simulink model "Redresseur_MLI_3Ph_2021_MLI_abc_s3b"  (R2022b)
settings: Solver=ode8  StartTime=0.0  StopTime=0.1  FixedStep=1e-6  RelTol=1e-3
undefined symbols (not defined in the file): C, Im, inverter_matrix, K, L, R, Ta, Td, Ti, V
libraries: simulink x1
settings Model: Creator=driss  LastModifiedBy=driss
settings RTWCC: GPUComputeCapability=5.0

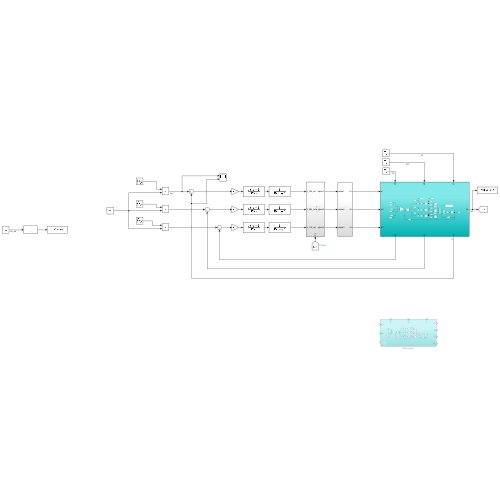
[thumbnail: Simulink's stored preview of the top-level diagram]
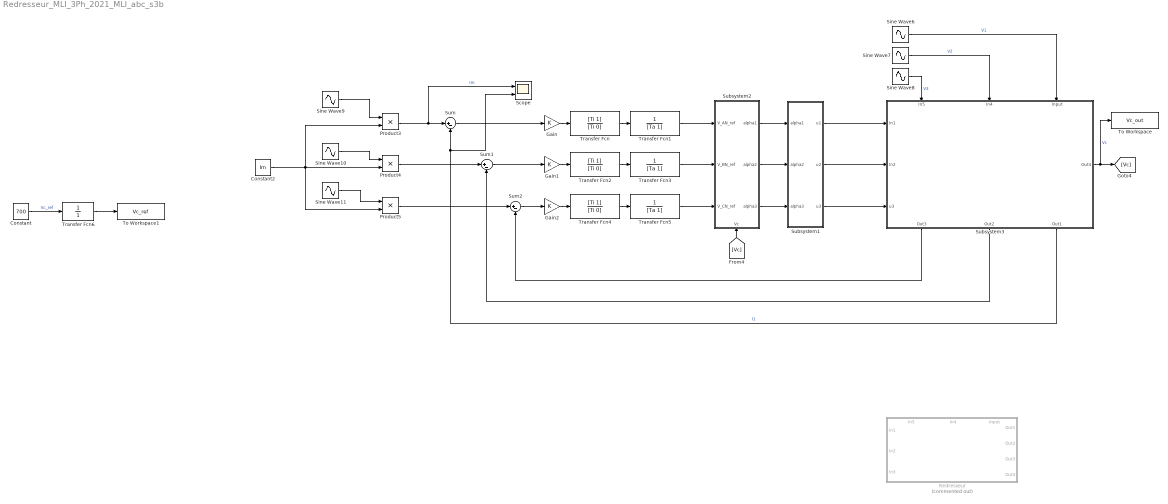
== system Redresseur_MLI_3Ph_2021_MLI_abc_s3b ==
  Constant : Constant  Value=700
  Constant2 : Constant  Value=Im
  Gain : Gain  Gain=K
  Gain1 : Gain  Gain=K
  Gain2 : Gain  Gain=K
  Product3 : Product
  Product4 : Product
  Product5 : Product
  Redresseur : Subsystem  Commented=on
      settings: PortSchema="{\"entries\":[{\"content\":{\"sides\":[{\"content\":{\"connectorIds\":[\"In1\",\"In2\",\"In3\"]},\"type\":\"ConnectorPlacement.EquallySpacedRectSide\",\"uuid\":\"ae9b6999-67aa-4d3c-bad5-5678f4aa6fd1\"},{\"content\":{\"connectorIds\":[\"Out1\",\"Out2\",\"Out3\",\"Out4\"],\"side\":\"RIGHT\"},\"type\":\"ConnectorPlacement.EquallySpacedRectSide\",\"uuid\":\"c2ea9883-df9a-4db0-b590-77b43908e459\"},{\"content\":{\"connectorIds\":[\"In4\",\"In5\",\"In6\"],\"side\":\"TOP\"},\"type\":\"ConnectorPlacement.EquallySpacedRectSide\",\"uuid\":\"cd2a08bf-72f9-4cdd-a271-8309bde71cde\"},{\"content\":{\"side\":\"BOTTOM\"},\"type\":\"ConnectorPlacement.EquallySpacedRectSide\",\"uuid\":\"317f1b40-2736-47c4-82a9-6da6172d899a\"}]},\"type\":\"ConnectorPlacement.EquallySpacedConnector\",\"uuid\":\"e059e48c-1350-41c9-95f4-730b69f1f213\"}],\"packageUris\":[\"http://schema.mathworks.com/mf0/Connector/R2020b\"],\"version\":\"1.0\"}"
  Scope : Scope  NumInputPorts=2
  Sine Wave10 : Sin  Frequency=2*50*pi  Phase=-2*pi/3  SampleTime=0
  Sine Wave11 : Sin  Frequency=2*50*pi  Phase=-4*pi/3  SampleTime=0
  Sine Wave6 : Sin  Amplitude=V*sqrt(2)  Frequency=2*50*pi  SampleTime=0
  Sine Wave7 : Sin  Amplitude=V*sqrt(2)  Frequency=2*50*pi  Phase=-2*pi/3  SampleTime=0
  Sine Wave8 : Sin  Amplitude=V*sqrt(2)  Frequency=2*50*pi  Phase=-4*pi/3  SampleTime=0
  Sine Wave9 : Sin  Frequency=2*50*pi  SampleTime=0
  Subsystem1 : Subsystem
  Subsystem2 : Subsystem
      settings: PortSchema="{\"entries\":[{\"content\":{\"sides\":[{\"content\":{\"connectorIds\":[\"In1\",\"In2\",\"In3\"]},\"type\":\"ConnectorPlacement.EquallySpacedRectSide\",\"uuid\":\"a3c0e225-73b1-4d6d-96ea-a79f2c69e987\"},{\"content\":{\"connectorIds\":[\"Out1\",\"Out2\",\"Out3\"],\"side\":\"RIGHT\"},\"type\":\"ConnectorPlacement.EquallySpacedRectSide\",\"uuid\":\"e47335df-8d84-45b3-8de3-f9ef23b68ce2\"},{\"content\":{\"connectorIds\":[],\"side\":\"TOP\"},\"type\":\"ConnectorPlacement.EquallySpacedRectSide\",\"uuid\":\"700b4ae9-e9d5-449c-823f-e97f4f733a61\"},{\"content\":{\"connectorIds\":[\"In4\"],\"side\":\"BOTTOM\"},\"type\":\"ConnectorPlacement.EquallySpacedRectSide\",\"uuid\":\"4332c11f-da0c-41da-94bc-63e1f62b18da\"}]},\"type\":\"ConnectorPlacement.EquallySpacedConnector\",\"uuid\":\"589f38f2-4ecb-4b26-afeb-66b253271d4e\"}],\"packageUris\":[\"http://schema.mathworks.com/mf0/Connector/R2020b\"],\"version\":\"1.0\"}"
  Subsystem3 : Subsystem
      settings: PortSchema="{\"entries\":[{\"content\":{\"sides\":[{\"content\":{\"connectorIds\":[\"In1\",\"In2\",\"In3\"]},\"type\":\"ConnectorPlacement.EquallySpacedRectSide\",\"uuid\":\"ae9b6999-67aa-4d3c-bad5-5678f4aa6fd1\"},{\"content\":{\"connectorIds\":[\"Out1\"],\"side\":\"RIGHT\"},\"type\":\"ConnectorPlacement.EquallySpacedRectSide\",\"uuid\":\"c2ea9883-df9a-4db0-b590-77b43908e459\"},{\"content\":{\"connectorIds\":[\"In4\",\"In5\",\"In6\"],\"side\":\"TOP\"},\"type\":\"ConnectorPlacement.EquallySpacedRectSide\",\"uuid\":\"cd2a08bf-72f9-4cdd-a271-8309bde71cde\"},{\"content\":{\"connectorIds\":[\"Out2\",\"Out3\",\"Out4\"],\"side\":\"BOTTOM\"},\"type\":\"ConnectorPlacement.EquallySpacedRectSide\",\"uuid\":\"317f1b40-2736-47c4-82a9-6da6172d899a\"}]},\"type\":\"ConnectorPlacement.EquallySpacedConnector\",\"uuid\":\"e059e48c-1350-41c9-95f4-730b69f1f213\"}],\"packageUris\":[\"http://schema.mathworks.com/mf0/Connector/R2020b\"],\"version\":\"1.0\"}"
  Sum : Sum  Inputs=|+-
  Sum1 : Sum  Inputs=|+-
  Sum2 : Sum  Inputs=|+-
  To Workspace : ToWorkspace  VariableName=Vc_out  SaveFormat=Timeseries  SampleTime=-1
  To Workspace1 : ToWorkspace  VariableName=Vc_ref  SaveFormat=Timeseries  SampleTime=-1
  Transfer Fcn : TransferFcn  Numerator=[Ti 1]  Denominator=[Ti 0]
  Transfer Fcn1 : TransferFcn  Denominator=[Ta 1]
  Transfer Fcn2 : TransferFcn  Numerator=[Ti 1]  Denominator=[Ti 0]
  Transfer Fcn3 : TransferFcn  Denominator=[Ta 1]
  Transfer Fcn4 : TransferFcn  Numerator=[Ti 1]  Denominator=[Ti 0]
  Transfer Fcn5 : TransferFcn  Denominator=[Ta 1]
  Transfer Fcn6 : TransferFcn  Denominator=[0 1]
  wires:
  Constant/1 -> Transfer Fcn6/1  "Vc_ref"
  Subsystem2/1(alpha1) -> Subsystem1/1(alpha1)
  Subsystem2/2(alpha2) -> Subsystem1/2(alpha2)
  Subsystem2/3(alpha3) -> Subsystem1/3(alpha3)
  Subsystem1/1(u1) -> Subsystem3/1(In1)
  Subsystem1/2(u2) -> Subsystem3/2(In2)
  Subsystem1/3(u3) -> Subsystem3/3(u3)
  Sine Wave7/1 -> Subsystem3/5(In4)  "V2"
  Sine Wave8/1 -> Subsystem3/4(In5)  "V3"
  Sine Wave6/1 -> Subsystem3/6(Input)  "V1"
  [Vc] -> Subsystem2/4(Vc)
  Subsystem3/1(Out4) -> To Workspace/1, [Vc]  "Vc"
  Sine Wave11/1 -> Product5/1
  Sine Wave10/1 -> Product4/1
  Sine Wave9/1 -> Product3/1
  Constant2/1 -> Product5/2, Product4/2, Product3/2
  Product3/1 -> Scope/1, Sum/1  "Im"
  Product4/1 -> Sum1/1
  Product5/1 -> Sum2/1
  Sum/1 -> Gain/1
  Gain/1 -> Transfer Fcn/1
  Transfer Fcn/1 -> Transfer Fcn1/1
  Transfer Fcn1/1 -> Subsystem2/1(V_AN_ref)
  Transfer Fcn2/1 -> Transfer Fcn3/1
  Gain1/1 -> Transfer Fcn2/1
  Transfer Fcn3/1 -> Subsystem2/2(V_BN_ref)
  Transfer Fcn5/1 -> Subsystem2/3(V_CN_ref)
  Gain2/1 -> Transfer Fcn4/1
  Transfer Fcn4/1 -> Transfer Fcn5/1
  Sum1/1 -> Gain1/1
  Sum2/1 -> Gain2/1
  Subsystem3/2(Out3) -> Sum2/2
  Subsystem3/3(Out2) -> Sum1/2
  Subsystem3/4(Out1) -> Scope/2, Sum/2  "I1"
  Transfer Fcn6/1 -> To Workspace1/1

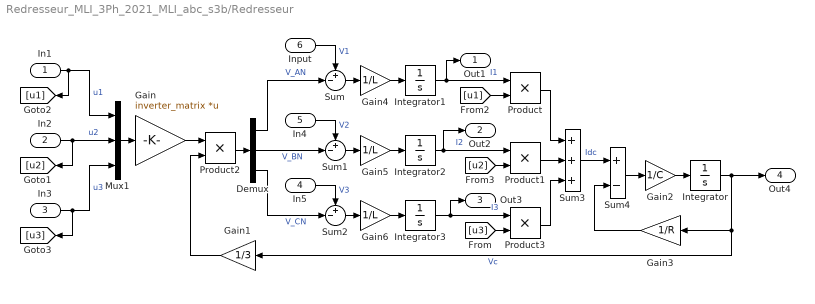
== system Redresseur_MLI_3Ph_2021_MLI_abc_s3b/Redresseur ==
  In1 : Inport
  In2 : Inport  Port=2
  In3 : Inport  Port=3
  In5 : Inport  Port=4
  In4 : Inport  Port=5
  Input : Inport  Port=6
  Demux : Demux  Outputs=3
  Gain : Gain  Gain=inverter_matrix  Multiplication=Matrix(K*u)
  Gain1 : Gain  Gain=1/3
  Gain2 : Gain  Gain=1/C
  Gain3 : Gain  Gain=1/R
  Gain4 : Gain  Gain=1/L
  Gain5 : Gain  Gain=1/L
  Gain6 : Gain  Gain=1/L
  Integrator{,1..3} (4 alike) : Integrator
  Mux1 : Mux  Inputs=3
  Product{,1..3} (4 alike) : Product
  Sum : Sum  Inputs=+-|
  Sum1 : Sum  Inputs=+-|
  Sum2 : Sum  Inputs=+-|
  Sum3 : Sum  Inputs=+++
  Sum4 : Sum  Inputs=+-
  Out1 : Outport
  Out2 : Outport  Port=2
  Out3 : Outport  Port=3
  Out4 : Outport  Port=4
  wires:
  In3/1 -> [u3], Mux1/3  "u3"
  In2/1 -> [u2], Mux1/2  "u2"
  In1/1 -> [u1], Mux1/1  "u1"
  Demux/2 -> Sum1/2  "V_BN"
  Demux/3 -> Sum2/2  "V_CN"
  Demux/1 -> Sum/2  "V_AN"
  Input/1 -> Sum/1  "V1"
  In4/1 -> Sum1/1  "V2"
  In5/1 -> Sum2/1  "V3"
  Sum/1 -> Gain4/1
  Sum1/1 -> Gain5/1
  Sum2/1 -> Gain6/1
  Integrator1/1 -> Out1/1, Product/1  "I1"
  Integrator3/1 -> Out3/1, Product3/1  "I3"
  Integrator2/1 -> Product1/1, Out2/1  "I2"
  Mux1/1 -> Gain/1
  [u3] -> Product3/2
  Product/1 -> Sum3/1
  Product1/1 -> Sum3/2
  Product3/1 -> Sum3/3
  Gain1/1 -> Product2/2
  Gain/1 -> Product2/1
  Sum3/1 -> Sum4/1  "Idc"
  Sum4/1 -> Gain2/1
  Gain2/1 -> Integrator/1
  Integrator/1 -> Out4/1, Gain1/1, Gain3/1  "Vc"
  Gain3/1 -> Sum4/2
  Gain4/1 -> Integrator1/1
  Gain5/1 -> Integrator2/1
  Gain6/1 -> Integrator3/1
  Product2/1 -> Demux/1
  [u1] -> Product/2
  [u2] -> Product1/2

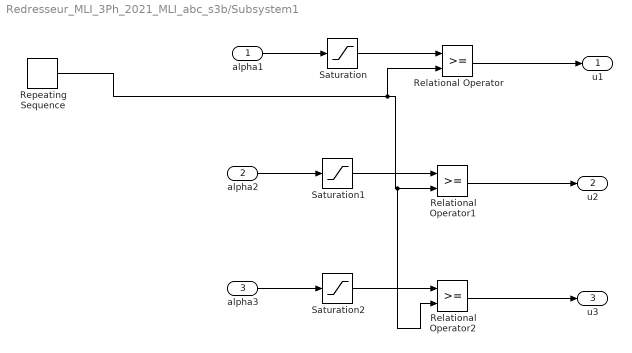
== system Redresseur_MLI_3Ph_2021_MLI_abc_s3b/Subsystem1 ==
  alpha1 : Inport
  alpha2 : Inport  Port=2
  alpha3 : Inport  Port=3
  Relational Operator : RelationalOperator  OutDataTypeStr=boolean  RndMeth=Simplest  InputSameDT=off
  Relational Operator1 : RelationalOperator  OutDataTypeStr=boolean  RndMeth=Simplest  InputSameDT=off
  Relational Operator2 : RelationalOperator  OutDataTypeStr=boolean  RndMeth=Simplest  InputSameDT=off
  Repeating Sequence : simulink/Sources/Repeating Sequence  rep_seq_t=[0 Td/2 Td]  rep_seq_y=[1 0 1]
  Saturation : Saturate  UpperLimit=1  LowerLimit=0
  Saturation1 : Saturate  UpperLimit=1  LowerLimit=0
  Saturation2 : Saturate  UpperLimit=1  LowerLimit=0
  u1 : Outport
  u2 : Outport  Port=2
  u3 : Outport  Port=3
  wires:
  Saturation/1 -> Relational Operator/1
  Relational Operator/1 -> u1/1
  alpha1/1 -> Saturation/1
  Saturation1/1 -> Relational Operator1/1
  Relational Operator1/1 -> u2/1
  alpha2/1 -> Saturation1/1
  Saturation2/1 -> Relational Operator2/1
  Relational Operator2/1 -> u3/1
  alpha3/1 -> Saturation2/1
  Repeating Sequence/1 -> Relational Operator2/2, Relational Operator1/2, Relational Operator/2

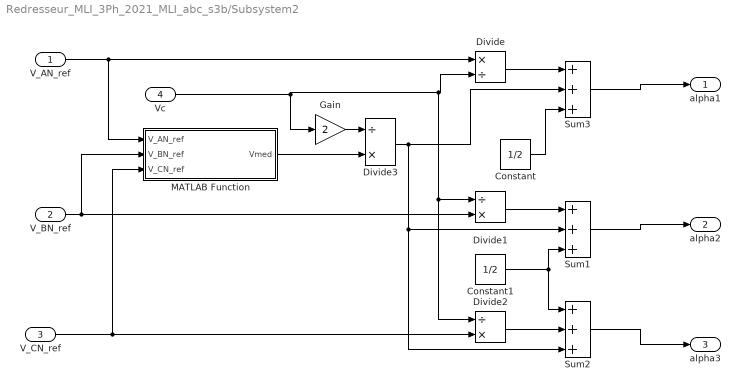
== system Redresseur_MLI_3Ph_2021_MLI_abc_s3b/Subsystem2 ==
  V_AN_ref : Inport
  V_BN_ref : Inport  Port=2
  V_CN_ref : Inport  Port=3
  Vc : Inport  Port=4
  Constant : Constant  Value=1/2
  Constant1 : Constant  Value=1/2
  Divide : Product  Inputs=*/
  Divide1 : Product  Inputs=/*
  Divide2 : Product  Inputs=/*
  Divide3 : Product  Inputs=/*
  Gain : Gain  Gain=2
  MATLAB Function : MATLAB Function  TreatAsAtomicUnit=on
  Sum1 : Sum  Inputs=+++
  Sum2 : Sum  Inputs=+++
  Sum3 : Sum  Inputs=+++
  alpha1 : Outport
  alpha2 : Outport  Port=2
  alpha3 : Outport  Port=3
  wires:
  Sum3/1 -> alpha1/1
  V_AN_ref/1 -> MATLAB Function/1(V_AN_ref), Divide/1
  Divide/1 -> Sum3/1
  Constant/1 -> Sum3/3
  MATLAB Function/1(Vmed) -> Divide3/2
  Gain/1 -> Divide3/1
  Constant1/1 -> Sum2/1, Sum1/3
  Sum1/1 -> alpha2/1
  Divide1/1 -> Sum1/1
  V_BN_ref/1 -> MATLAB Function/2(V_BN_ref), Divide1/2
  Divide3/1 -> Sum2/3, Sum1/2, Sum3/2
  Vc/1 -> Divide2/1, Divide1/1, Divide/2, Gain/1
  V_CN_ref/1 -> Divide2/2, MATLAB Function/3(V_CN_ref)
  Divide2/1 -> Sum2/2
  Sum2/1 -> alpha3/1

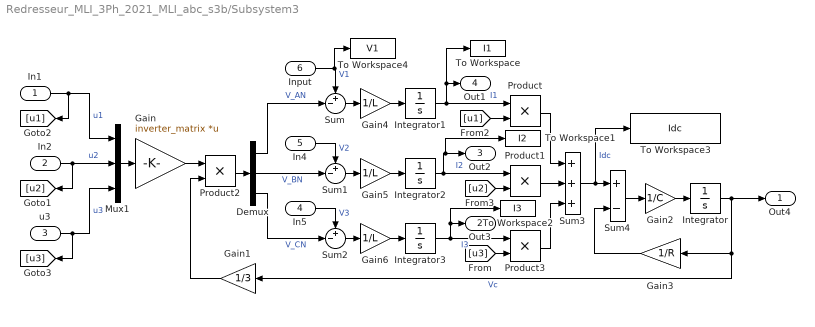
== system Redresseur_MLI_3Ph_2021_MLI_abc_s3b/Subsystem3 ==
  In1 : Inport
  In2 : Inport  Port=2
  u3 : Inport  Port=3
  In5 : Inport  Port=4
  In4 : Inport  Port=5
  Input : Inport  Port=6
  Demux : Demux  Outputs=3
  Gain : Gain  Gain=inverter_matrix  Multiplication=Matrix(K*u)
  Gain1 : Gain  Gain=1/3
  Gain2 : Gain  Gain=1/C
  Gain3 : Gain  Gain=1/R
  Gain4 : Gain  Gain=1/L
  Gain5 : Gain  Gain=1/L
  Gain6 : Gain  Gain=1/L
  Integrator : Integrator  InitialCondition=1  LimitOutput=on  LowerSaturationLimit=0
  Integrator1 : Integrator
  Integrator2 : Integrator
  Integrator3 : Integrator
  Mux1 : Mux  Inputs=3
  Product{,1..3} (4 alike) : Product
  Sum : Sum  Inputs=+-|
  Sum1 : Sum  Inputs=+-|
  Sum2 : Sum  Inputs=+-|
  Sum3 : Sum  Inputs=+++
  Sum4 : Sum  Inputs=+-
  To Workspace : ToWorkspace  VariableName=I1  SaveFormat=Timeseries  SampleTime=-1
  To Workspace1 : ToWorkspace  VariableName=I2  SaveFormat=Timeseries  SampleTime=-1
  To Workspace2 : ToWorkspace  VariableName=I3  SaveFormat=Timeseries  SampleTime=-1
  To Workspace3 : ToWorkspace  VariableName=Idc  SaveFormat=Timeseries  SampleTime=-1
  To Workspace4 : ToWorkspace  VariableName=V1  SaveFormat=Timeseries  SampleTime=-1
  Out4 : Outport
  Out3 : Outport  Port=2
  Out2 : Outport  Port=3
  Out1 : Outport  Port=4
  wires:
  [u2] -> Product1/2
  [u1] -> Product/2
  Product2/1 -> Demux/1
  Gain6/1 -> Integrator3/1
  Gain5/1 -> Integrator2/1
  Gain4/1 -> Integrator1/1
  Gain3/1 -> Sum4/2
  Integrator/1 -> Gain3/1, Gain1/1, Out4/1  "Vc"
  Gain2/1 -> Integrator/1
  Sum4/1 -> Gain2/1
  Sum3/1 -> Sum4/1, To Workspace3/1  "Idc"
  Gain/1 -> Product2/1
  Gain1/1 -> Product2/2
  Product3/1 -> Sum3/3
  Product1/1 -> Sum3/2
  Product/1 -> Sum3/1
  [u3] -> Product3/2
  Mux1/1 -> Gain/1
  Integrator2/1 -> Out2/1, To Workspace1/1, Product1/1  "I2"
  Integrator3/1 -> Product3/1, Out3/1, To Workspace2/1  "I3"
  Integrator1/1 -> Product/1, Out1/1, To Workspace/1  "I1"
  Sum2/1 -> Gain6/1
  Sum1/1 -> Gain5/1
  Sum/1 -> Gain4/1
  In5/1 -> Sum2/1  "V3"
  In4/1 -> Sum1/1  "V2"
  Input/1 -> Sum/1, To Workspace4/1  "V1"
  Demux/1 -> Sum/2  "V_AN"
  Demux/3 -> Sum2/2  "V_CN"
  Demux/2 -> Sum1/2  "V_BN"
  In1/1 -> Mux1/1, [u1]  "u1"
  In2/1 -> Mux1/2, [u2]  "u2"
  u3/1 -> Mux1/3, [u3]  "u3"

== matlab function Redresseur_MLI_3Ph_2021_MLI_abc_s3b/Subsystem2/MATLAB Function ==
  data: V_AN_ref input; Vmed output; V_BN_ref input; V_CN_ref input
function Vmed = fcn(V_AN_ref,V_BN_ref,V_CN_ref)
     V_set = [V_AN_ref V_BN_ref V_CN_ref];
Vmed= -(min(V_set) + max(V_set));
